simulink model "MultiIntersectionStoplight"  (R2020a)
settings: Solver=VariableStepAuto  StartTime=0.0  StopTime=inf  RelTol=1e-3
libraries: dspnetwork x63, sldrtlib x1
settings Model: Creator=brandon  LastModifiedBy=brandon

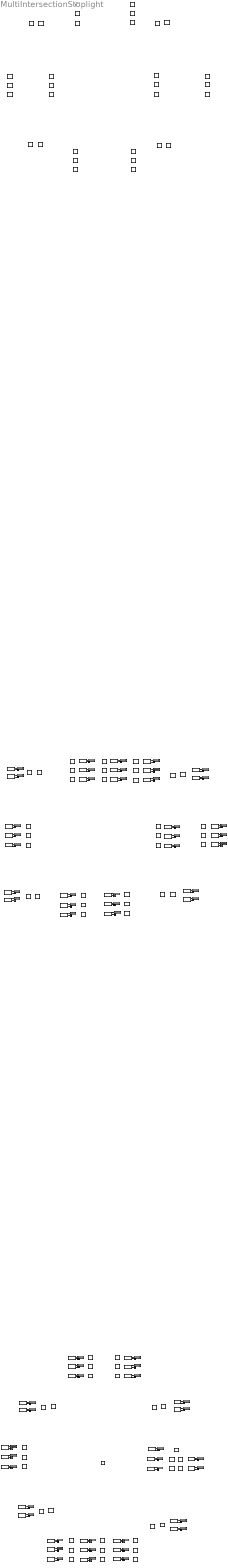
== system MultiIntersectionStoplight ==
  note: Walk: UDP 25001
      | Don't Walk: UDP 25002
  note: Walk: UDP 25003
      | Don't Walk: UDP 25004
  note: Walk: UDP 25005
      | Don't Walk: UDP 25006
  note: Walk: UDP 25007
      | Don't Walk: UDP 25008
  note: Red: UDP 26001
      | Yellow: UDP 26002
      | Green: UDP 26003
  note: Red: UDP 26004
      | Yellow: UDP 26005
      | Green: UDP 26006
  note: Red: UDP 26007
      | Yellow: UDP 26008
      | Green: UDP 26009
  note: Red: UDP 26010
      | Yellow: UDP 26011
      | Green: UDP 26012
  note: Red: UDP 26013
      | Yellow: UDP 26014
      | Green: UDP 26015
  note: Red: UDP 26016
      | Yellow: UDP 26017
      | Green: UDP 26018
  note: Red: UDP 26019
      | Yellow: UDP 26020
      | Green: UDP 26021
      | Yellow Left: UDP 26022
      | Green Left: UDP 26023
  Display{1..63} (63 alike) : Display
  Lamp{12..106} (95 alike) : LampBlock  LabelPosition=Hide
  Real-Time Synchronization : sldrtlib/Real-Time Synchronization  SampleTime=0.1  MaxMissedTicks=1000000  ShowMissedTicks=off  YieldWhenWaiting=off
  Terminator{1..63} (63 alike) : Terminator
  UDP Receive1 : dspnetwork/UDP Receive  localURL='0.0.0.0'  localPort=26010  remoteURL='0.0.0.0'  remotePort=-1  recvBufferSize=2  dims=1  signalDatatype=uint16  isComplex=off  isVarSize=off  showBlockingTime=off  blockingTime=0  sampletime=0.1  blockPlatform=[]
  UDP Receive10 : dspnetwork/UDP Receive  localURL='0.0.0.0'  localPort=26016  remoteURL='0.0.0.0'  remotePort=-1  recvBufferSize=2  dims=1  signalDatatype=uint16  isComplex=off  isVarSize=off  showBlockingTime=off  blockingTime=0  sampletime=0.1  blockPlatform=[]
  UDP Receive11 : dspnetwork/UDP Receive  localURL='0.0.0.0'  localPort=26013  remoteURL='0.0.0.0'  remotePort=-1  recvBufferSize=2  dims=1  signalDatatype=uint16  isComplex=off  isVarSize=off  showBlockingTime=off  blockingTime=0  sampletime=0.1  blockPlatform=[]
  UDP Receive12 : dspnetwork/UDP Receive  localURL='0.0.0.0'  localPort=26007  remoteURL='0.0.0.0'  remotePort=-1  recvBufferSize=2  dims=1  signalDatatype=uint16  isComplex=off  isVarSize=off  showBlockingTime=off  blockingTime=0  sampletime=0.1  blockPlatform=[]
  UDP Receive13 : dspnetwork/UDP Receive  localURL='0.0.0.0'  localPort=26008  remoteURL='0.0.0.0'  remotePort=-1  recvBufferSize=2  dims=1  signalDatatype=uint16  isComplex=off  isVarSize=off  showBlockingTime=off  blockingTime=0  sampletime=0.1  blockPlatform=[]
  UDP Receive14 : dspnetwork/UDP Receive  localURL='0.0.0.0'  localPort=26009  remoteURL='0.0.0.0'  remotePort=-1  recvBufferSize=2  dims=1  signalDatatype=uint16  isComplex=off  isVarSize=off  showBlockingTime=off  blockingTime=0  sampletime=0.1  blockPlatform=[]
  UDP Receive15 : dspnetwork/UDP Receive  localURL='0.0.0.0'  localPort=26004  remoteURL='0.0.0.0'  remotePort=-1  recvBufferSize=2  dims=1  signalDatatype=uint16  isComplex=off  isVarSize=off  showBlockingTime=off  blockingTime=0  sampletime=0.1  blockPlatform=[]
  UDP Receive16 : dspnetwork/UDP Receive  localURL='0.0.0.0'  localPort=26005  remoteURL='0.0.0.0'  remotePort=-1  recvBufferSize=2  dims=1  signalDatatype=uint16  isComplex=off  isVarSize=off  showBlockingTime=off  blockingTime=0  sampletime=0.1  blockPlatform=[]
  UDP Receive17 : dspnetwork/UDP Receive  localURL='0.0.0.0'  localPort=26006  remoteURL='0.0.0.0'  remotePort=-1  recvBufferSize=2  dims=1  signalDatatype=uint16  isComplex=off  isVarSize=off  showBlockingTime=off  blockingTime=0  sampletime=0.1  blockPlatform=[]
  UDP Receive18 : dspnetwork/UDP Receive  localURL='0.0.0.0'  localPort=26001  remoteURL='0.0.0.0'  remotePort=-1  recvBufferSize=2  dims=1  signalDatatype=uint16  isComplex=off  isVarSize=off  showBlockingTime=off  blockingTime=0  sampletime=0.1  blockPlatform=[]
  UDP Receive19 : dspnetwork/UDP Receive  localURL='0.0.0.0'  localPort=26002  remoteURL='0.0.0.0'  remotePort=-1  recvBufferSize=2  dims=1  signalDatatype=uint16  isComplex=off  isVarSize=off  showBlockingTime=off  blockingTime=0  sampletime=0.1  blockPlatform=[]
  UDP Receive2 : dspnetwork/UDP Receive  localURL='0.0.0.0'  localPort=26011  remoteURL='0.0.0.0'  remotePort=-1  recvBufferSize=2  dims=1  signalDatatype=uint16  isComplex=off  isVarSize=off  showBlockingTime=off  blockingTime=0  sampletime=0.1  blockPlatform=[]
  UDP Receive20 : dspnetwork/UDP Receive  localURL='0.0.0.0'  localPort=26003  remoteURL='0.0.0.0'  remotePort=-1  recvBufferSize=2  dims=1  signalDatatype=uint16  isComplex=off  isVarSize=off  showBlockingTime=off  blockingTime=0  sampletime=0.1  blockPlatform=[]
  UDP Receive{21,32..63} (33 alike) : dspnetwork/UDP Receive  localURL='0.0.0.0'  localPort=25003  remoteURL='0.0.0.0'  remotePort=-1  recvBufferSize=2  dims=1  signalDatatype=uint16  isComplex=off  isVarSize=off  showBlockingTime=off  blockingTime=0  sampletime=0.1  blockPlatform=[]
  UDP Receive22 : dspnetwork/UDP Receive  localURL='0.0.0.0'  localPort=25004  remoteURL='0.0.0.0'  remotePort=-1  recvBufferSize=2  dims=1  signalDatatype=uint16  isComplex=off  isVarSize=off  showBlockingTime=off  blockingTime=0  sampletime=0.1  blockPlatform=[]
  UDP Receive23 : dspnetwork/UDP Receive  localURL='0.0.0.0'  localPort=25001  remoteURL='0.0.0.0'  remotePort=-1  recvBufferSize=2  dims=1  signalDatatype=uint16  isComplex=off  isVarSize=off  showBlockingTime=off  blockingTime=0  sampletime=0.1  blockPlatform=[]
  UDP Receive24 : dspnetwork/UDP Receive  localURL='0.0.0.0'  localPort=25002  remoteURL='0.0.0.0'  remotePort=-1  recvBufferSize=2  dims=1  signalDatatype=uint16  isComplex=off  isVarSize=off  showBlockingTime=off  blockingTime=0  sampletime=0.1  blockPlatform=[]
  UDP Receive25 : dspnetwork/UDP Receive  localURL='0.0.0.0'  localPort=26021  remoteURL='0.0.0.0'  remotePort=-1  recvBufferSize=2  dims=1  signalDatatype=uint16  isComplex=off  isVarSize=off  showBlockingTime=off  blockingTime=0  sampletime=0.1  blockPlatform=[]
  UDP Receive26 : dspnetwork/UDP Receive  localURL='0.0.0.0'  localPort=26020  remoteURL='0.0.0.0'  remotePort=-1  recvBufferSize=2  dims=1  signalDatatype=uint16  isComplex=off  isVarSize=off  showBlockingTime=off  blockingTime=0  sampletime=0.1  blockPlatform=[]
  UDP Receive27 : dspnetwork/UDP Receive  localURL='0.0.0.0'  localPort=26023  remoteURL='0.0.0.0'  remotePort=-1  recvBufferSize=2  dims=1  signalDatatype=uint16  isComplex=off  isVarSize=off  showBlockingTime=off  blockingTime=0  sampletime=0.1  blockPlatform=[]
  UDP Receive28 : dspnetwork/UDP Receive  localURL='0.0.0.0'  localPort=26022  remoteURL='0.0.0.0'  remotePort=-1  recvBufferSize=2  dims=1  signalDatatype=uint16  isComplex=off  isVarSize=off  showBlockingTime=off  blockingTime=0  sampletime=0.1  blockPlatform=[]
  UDP Receive29 : dspnetwork/UDP Receive  localURL='0.0.0.0'  localPort=26019  remoteURL='0.0.0.0'  remotePort=-1  recvBufferSize=2  dims=1  signalDatatype=uint16  isComplex=off  isVarSize=off  showBlockingTime=off  blockingTime=0  sampletime=0.1  blockPlatform=[]
  UDP Receive3 : dspnetwork/UDP Receive  localURL='0.0.0.0'  localPort=25007  remoteURL='0.0.0.0'  remotePort=-1  recvBufferSize=2  dims=1  signalDatatype=uint16  isComplex=off  isVarSize=off  showBlockingTime=off  blockingTime=0  sampletime=0.1  blockPlatform=[]
  UDP Receive30 : dspnetwork/UDP Receive  localURL='0.0.0.0'  localPort=26014  remoteURL='0.0.0.0'  remotePort=-1  recvBufferSize=2  dims=1  signalDatatype=uint16  isComplex=off  isVarSize=off  showBlockingTime=off  blockingTime=0  sampletime=0.1  blockPlatform=[]
  UDP Receive31 : dspnetwork/UDP Receive  localURL='0.0.0.0'  localPort=26015  remoteURL='0.0.0.0'  remotePort=-1  recvBufferSize=2  dims=1  signalDatatype=uint16  isComplex=off  isVarSize=off  showBlockingTime=off  blockingTime=0  sampletime=0.1  blockPlatform=[]
  UDP Receive4 : dspnetwork/UDP Receive  localURL='0.0.0.0'  localPort=25008  remoteURL='0.0.0.0'  remotePort=-1  recvBufferSize=2  dims=1  signalDatatype=uint16  isComplex=off  isVarSize=off  showBlockingTime=off  blockingTime=0  sampletime=0.1  blockPlatform=[]
  UDP Receive5 : dspnetwork/UDP Receive  localURL='0.0.0.0'  localPort=26018  remoteURL='0.0.0.0'  remotePort=-1  recvBufferSize=2  dims=1  signalDatatype=uint16  isComplex=off  isVarSize=off  showBlockingTime=off  blockingTime=0  sampletime=0.1  blockPlatform=[]
  UDP Receive6 : dspnetwork/UDP Receive  localURL='0.0.0.0'  localPort=26012  remoteURL='0.0.0.0'  remotePort=-1  recvBufferSize=2  dims=1  signalDatatype=uint16  isComplex=off  isVarSize=off  showBlockingTime=off  blockingTime=0  sampletime=0.1  blockPlatform=[]
  UDP Receive7 : dspnetwork/UDP Receive  localURL='0.0.0.0'  localPort=25006  remoteURL='0.0.0.0'  remotePort=-1  recvBufferSize=2  dims=1  signalDatatype=uint16  isComplex=off  isVarSize=off  showBlockingTime=off  blockingTime=0  sampletime=0.1  blockPlatform=[]
  UDP Receive8 : dspnetwork/UDP Receive  localURL='0.0.0.0'  localPort=25005  remoteURL='0.0.0.0'  remotePort=-1  recvBufferSize=2  dims=1  signalDatatype=uint16  isComplex=off  isVarSize=off  showBlockingTime=off  blockingTime=0  sampletime=0.1  blockPlatform=[]
  UDP Receive9 : dspnetwork/UDP Receive  localURL='0.0.0.0'  localPort=26017  remoteURL='0.0.0.0'  remotePort=-1  recvBufferSize=2  dims=1  signalDatatype=uint16  isComplex=off  isVarSize=off  showBlockingTime=off  blockingTime=0  sampletime=0.1  blockPlatform=[]
  wires:
  UDP Receive12/1 -> Display12/1
  UDP Receive12/2 -> Terminator12/1
  UDP Receive13/2 -> Terminator13/1
  UDP Receive13/1 -> Display13/1
  UDP Receive14/2 -> Terminator14/1
  UDP Receive14/1 -> Display14/1
  UDP Receive15/2 -> Terminator15/1
  UDP Receive15/1 -> Display15/1
  UDP Receive16/2 -> Terminator16/1
  UDP Receive16/1 -> Display16/1
  UDP Receive17/2 -> Terminator17/1
  UDP Receive17/1 -> Display17/1
  UDP Receive18/2 -> Terminator18/1
  UDP Receive18/1 -> Display18/1
  UDP Receive19/2 -> Terminator19/1
  UDP Receive19/1 -> Display19/1
  UDP Receive20/2 -> Terminator20/1
  UDP Receive20/1 -> Display20/1
  UDP Receive21/2 -> Terminator21/1
  UDP Receive21/1 -> Display21/1
  UDP Receive22/2 -> Terminator22/1
  UDP Receive22/1 -> Display22/1
  UDP Receive23/2 -> Terminator23/1
  UDP Receive23/1 -> Display23/1
  UDP Receive24/2 -> Terminator24/1
  UDP Receive24/1 -> Display24/1
  UDP Receive25/2 -> Terminator25/1
  UDP Receive25/1 -> Display25/1
  UDP Receive26/2 -> Terminator26/1
  UDP Receive26/1 -> Display26/1
  UDP Receive27/2 -> Terminator27/1
  UDP Receive27/1 -> Display27/1
  UDP Receive28/2 -> Terminator28/1
  UDP Receive28/1 -> Display28/1
  UDP Receive29/2 -> Terminator29/1
  UDP Receive29/1 -> Display29/1
  UDP Receive1/2 -> Terminator1/1
  UDP Receive1/1 -> Display1/1
  UDP Receive2/2 -> Terminator2/1
  UDP Receive2/1 -> Display2/1
  UDP Receive6/2 -> Terminator6/1
  UDP Receive6/1 -> Display6/1
  UDP Receive7/2 -> Terminator7/1
  UDP Receive7/1 -> Display7/1
  UDP Receive8/2 -> Terminator8/1
  UDP Receive8/1 -> Display8/1
  UDP Receive3/2 -> Terminator3/1
  UDP Receive3/1 -> Display3/1
  UDP Receive4/2 -> Terminator4/1
  UDP Receive4/1 -> Display4/1
  UDP Receive5/2 -> Terminator5/1
  UDP Receive5/1 -> Display5/1
  UDP Receive9/2 -> Terminator9/1
  UDP Receive9/1 -> Display9/1
  UDP Receive10/2 -> Terminator10/1
  UDP Receive10/1 -> Display10/1
  UDP Receive11/2 -> Terminator11/1
  UDP Receive11/1 -> Display11/1
  UDP Receive30/2 -> Terminator30/1
  UDP Receive30/1 -> Display30/1
  UDP Receive31/2 -> Terminator31/1
  UDP Receive31/1 -> Display31/1
  UDP Receive32/2 -> Terminator32/1
  UDP Receive32/1 -> Display32/1
  UDP Receive33/2 -> Terminator33/1
  UDP Receive33/1 -> Display33/1
  UDP Receive34/2 -> Terminator34/1
  UDP Receive34/1 -> Display34/1
  UDP Receive35/2 -> Terminator35/1
  UDP Receive35/1 -> Display35/1
  UDP Receive36/2 -> Terminator36/1
  UDP Receive36/1 -> Display36/1
  UDP Receive37/2 -> Terminator37/1
  UDP Receive37/1 -> Display37/1
  UDP Receive38/2 -> Terminator38/1
  UDP Receive38/1 -> Display38/1
  UDP Receive39/2 -> Terminator39/1
  UDP Receive39/1 -> Display39/1
  UDP Receive40/2 -> Terminator40/1
  UDP Receive40/1 -> Display40/1
  UDP Receive41/2 -> Terminator41/1
  UDP Receive41/1 -> Display41/1
  UDP Receive42/2 -> Terminator42/1
  UDP Receive42/1 -> Display42/1
  UDP Receive43/2 -> Terminator43/1
  UDP Receive43/1 -> Display43/1
  UDP Receive44/2 -> Terminator44/1
  UDP Receive44/1 -> Display44/1
  UDP Receive45/2 -> Terminator45/1
  UDP Receive45/1 -> Display45/1
  UDP Receive46/2 -> Terminator46/1
  UDP Receive46/1 -> Display46/1
  UDP Receive47/2 -> Terminator47/1
  UDP Receive47/1 -> Display47/1
  UDP Receive48/2 -> Terminator48/1
  UDP Receive48/1 -> Display48/1
  UDP Receive49/2 -> Terminator49/1
  UDP Receive49/1 -> Display49/1
  UDP Receive50/2 -> Terminator50/1
  UDP Receive50/1 -> Display50/1
  UDP Receive51/2 -> Terminator51/1
  UDP Receive51/1 -> Display51/1
  UDP Receive52/2 -> Terminator52/1
  UDP Receive52/1 -> Display52/1
  UDP Receive53/2 -> Terminator53/1
  UDP Receive53/1 -> Display53/1
  UDP Receive54/2 -> Terminator54/1
  UDP Receive54/1 -> Display54/1
  UDP Receive55/2 -> Terminator55/1
  UDP Receive55/1 -> Display55/1
  UDP Receive56/2 -> Terminator56/1
  UDP Receive56/1 -> Display56/1
  UDP Receive57/2 -> Terminator57/1
  UDP Receive57/1 -> Display57/1
  UDP Receive58/2 -> Terminator58/1
  UDP Receive58/1 -> Display58/1
  UDP Receive59/2 -> Terminator59/1
  UDP Receive59/1 -> Display59/1
  UDP Receive60/2 -> Terminator60/1
  UDP Receive60/1 -> Display60/1
  UDP Receive61/2 -> Terminator61/1
  UDP Receive61/1 -> Display61/1
  UDP Receive62/2 -> Terminator62/1
  UDP Receive62/1 -> Display62/1
  UDP Receive63/2 -> Terminator63/1
  UDP Receive63/1 -> Display63/1
